simulink model "filtr_zerujacy"  (R2018a)
settings: Solver=VariableStepAuto  StartTime=0.0  StopTime=0.05  RelTol=1e-3
undefined symbols (not defined in the file): Ts
settings Model: Creator=klukomski  LastModifiedBy=klukomski

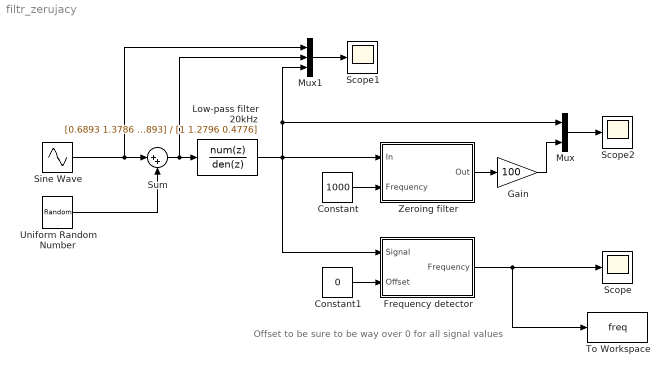
== system filtr_zerujacy ==
  note: Offset to be sure to be way over 0 for all signal values
  Constant : Constant  Value=1000
  Constant1 : Constant  Value=0
  Frequency detector : Subsystem
  Gain : Gain  Gain=100
  Low-pass filter 20kHz : DiscreteFilter  Numerator=[0.6893 1.3786 0.6893]  Denominator=[1 1.2796 0.4776]
  Mux : Mux  Inputs=2
  Mux1 : Mux  Inputs=3
  Scope : Scope
  Scope1 : Scope
  Scope2 : Scope
  Sine Wave : Sin  Bias=2  Frequency=2*pi*1000  SampleTime=0
  Sum : Sum  Inputs=|++
  To Workspace : ToWorkspace  VariableName=freq  SaveFormat=Timeseries  SampleTime=-1
  Uniform Random Number : UniformRandomNumber  Minimum=-0.1  Maximum=0.1  SampleTime=Ts*3
  Zeroing filter : Subsystem
  wires:
  Frequency detector/1(Frequency) -> To Workspace/1, Scope/1
  Constant/1 -> Zeroing filter/2(Frequency)
  Mux/1 -> Scope2/1
  Constant1/1 -> Frequency detector/2(Offset)
  Zeroing filter/1(Out) -> Gain/1
  Gain/1 -> Mux/2
  Sine Wave/1 -> Mux1/1, Sum/1
  Mux1/1 -> Scope1/1
  Uniform Random Number/1 -> Sum/2
  Sum/1 -> Mux1/2, Low-pass filter 20kHz/1
  Low-pass filter 20kHz/1 -> Frequency detector/1(Signal), Mux/1, Mux1/3, Zeroing filter/1(In)

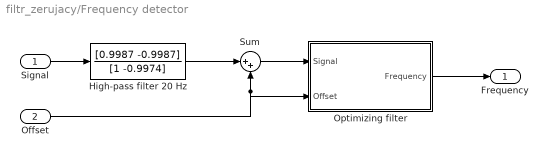
== system filtr_zerujacy/Frequency detector ==
  Signal : Inport
  Offset : Inport  Port=2
  High-pass filter 20 Hz : DiscreteFilter  Numerator=[0.9987 -0.9987]  Denominator=[1 -0.9974]  SampleTime=Ts
  Optimizing filter : Subsystem
  Sum : Sum  Inputs=|++
  Frequency : Outport
  wires:
  Offset/1 -> Sum/2, Optimizing filter/2(Offset)
  Optimizing filter/1(Frequency) -> Frequency/1
  Signal/1 -> High-pass filter 20 Hz/1
  High-pass filter 20 Hz/1 -> Sum/1
  Sum/1 -> Optimizing filter/1(Signal)

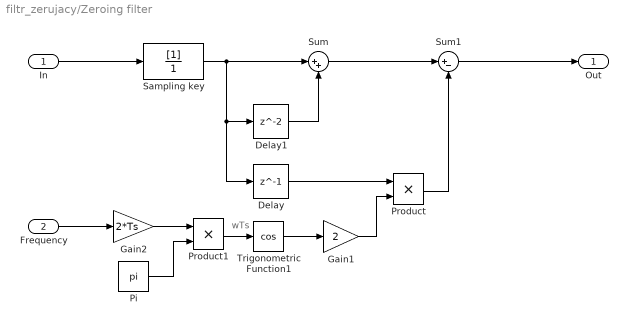
== system filtr_zerujacy/Zeroing filter ==
  note: wTs
  In : Inport
  Frequency : Inport  Port=2
  Delay : Delay  DelayLength=1  SampleTime=Ts
  Delay1 : Delay  SampleTime=Ts
  Gain1 : Gain  Gain=2
  Gain2 : Gain  Gain=2*Ts
  Pi : Constant  Value=pi
  Product : Product
  Product1 : Product
  Sampling key : DiscreteFilter  Denominator=1  SampleTime=Ts
  Sum : Sum  Inputs=|++
  Sum1 : Sum  Inputs=|+-
  Trigonometric Function1 : Trigonometry  Operator=cos
  Out : Outport
  wires:
  Delay1/1 -> Sum/2
  In/1 -> Sampling key/1
  Sampling key/1 -> Sum/1, Delay/1, Delay1/1
  Frequency/1 -> Gain2/1
  Trigonometric Function1/1 -> Gain1/1
  Gain1/1 -> Product/2
  Product1/1 -> Trigonometric Function1/1
  Gain2/1 -> Product1/1
  Pi/1 -> Product1/2
  Delay/1 -> Product/1
  Sum/1 -> Sum1/1
  Sum1/1 -> Out/1
  Product/1 -> Sum1/2

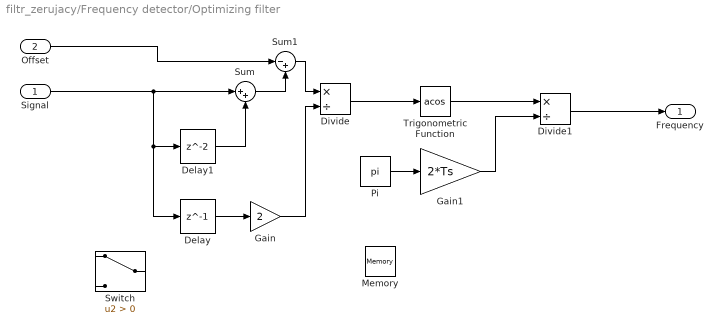
== system filtr_zerujacy/Frequency detector/Optimizing filter ==
  Signal : Inport
  Offset : Inport  Port=2
  Delay : Delay  DelayLength=1  SampleTime=Ts
  Delay1 : Delay  SampleTime=Ts
  Divide : Product  Inputs=*/
  Divide1 : Product  Inputs=*/
  Gain : Gain  Gain=2
  Gain1 : Gain  Gain=2*Ts
  Memory : Memory
  Pi : Constant  Value=pi
  Sum : Sum  Inputs=|++
  Sum1 : Sum  Inputs=|-+
  Switch : Switch  Criteria=u2 > Threshold
  Trigonometric Function : Trigonometry  Operator=acos
  Frequency : Outport
  wires:
  Delay/1 -> Gain/1
  Gain/1 -> Divide/2
  Signal/1 -> Sum/1, Delay1/1, Delay/1
  Delay1/1 -> Sum/2
  Trigonometric Function/1 -> Divide1/1
  Divide1/1 -> Frequency/1
  Pi/1 -> Gain1/1
  Sum1/1 -> Divide/1
  Gain1/1 -> Divide1/2
  Divide/1 -> Trigonometric Function/1
  Offset/1 -> Sum1/1
  Sum/1 -> Sum1/2
